simulink model "p2"  (R2024b)
settings: Solver=VariableStepAuto  StartTime=0.0  StopTime=0.7  RelTol=1e-3
settings Model: Creator=dunca  LastModifiedBy=Denis
settings RTWCC: GPUComputeCapability=3.5

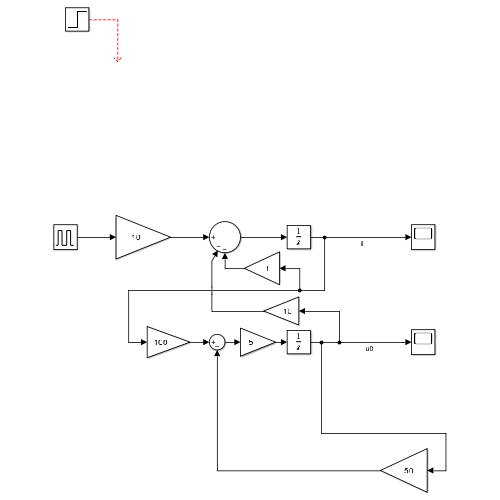
[thumbnail: Simulink's stored preview of the top-level diagram]
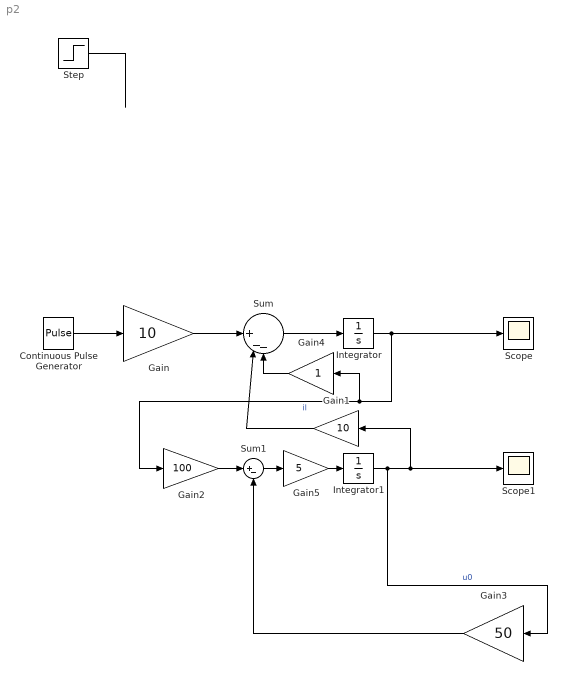
== system p2 ==
  Continuous Pulse Generator : DiscretePulseGenerator  PulseType=Time based  Amplitude=24  Period=1/23  PulseWidth=50
  Gain : Gain  Gain=10
  Gain1 : Gain  Gain=10
  Gain2 : Gain  Gain=100
  Gain3 : Gain  Gain=50
  Gain4 : Gain
  Gain5 : Gain  Gain=5
  Integrator : Integrator
  Integrator1 : Integrator
  Scope : Scope
  Scope1 : Scope
  Step : Step  Time=0.2  After=12  SampleTime=0
  Sum : Sum  Inputs=|||+|--
  Sum1 : Sum  Inputs=|+-
  wires:
  Gain2/1 -> Sum1/1
  Gain1/1 -> Sum/2
  Integrator/1 -> Gain4/1, Gain2/1, Scope/1  "il"
  Gain/1 -> Sum/1
  Integrator1/1 -> Gain3/1, Scope1/1, Gain1/1  "u0"
  Sum/1 -> Integrator/1
  Sum1/1 -> Gain5/1
  Gain3/1 -> Sum1/2
  Gain4/1 -> Sum/3
  Gain5/1 -> Integrator1/1
  Step/1 -> ?
  Continuous Pulse Generator/1 -> Gain/1
